simulink model "FullCardioLabModel"  (R2023b)
settings: Solver=FixedStepDiscrete  StartTime=0.0  StopTime=param_sim_time  FixedStep=1/fs  MaxStep=1/fs  RelTol=1e-3
undefined symbols (not defined in the file): analyses, fdesignblkfcn, fs, gcbh, param_tot_samples
libraries: dspstat3 x13, SCGAnalysis_SignalGenerationLib x2
(part 4 of 20)

== system FullCardioLabModel/ECG Preprocessing/Enabled ECG Preprocessing Subsystem/ECG Filtfiltering/Bandpass Filter 2 ==
  In : Inport
  Generated Filter Block : DiscreteFir  Tag=BlockMethodSubSystem  Coefficients=[-0.00679485432608760258 -0.00368052369966220989 0.00854312547844450834 -0.00080100055038292311 0.00372672989233903233 -0.000414423493004983272 0.00116500696533589489 -0.00068747703460298674 -0.00013687627970678594 -0.000908036536334603768 -0.000644757715485386033 -0.000872603667353300666 -0.000649980563873023558 -0.000610089182523331809 -0.00038439095041600032 -0.00024106878235529626 -4.03649627099907346e-05 0.000102557079219553864 0.000239825065708428893 0.000323758429883300614 0.000376057404680168019 0.000381073126084808557 0.000351986827882749646 0.000288970153653461583 0.000203557617554966464 0.000103021925348629849 -2.14972891546076422e-06 -0.000103131395606973747 -0.000191913507308220108 -0.000261698858359729039 -0.000308472416490167939 -0.000329303004746908082 -0.000324728524771220875 -0.000295994179250205389 -0.000247522226025559291 -0.000183683342227257597 -0.000111268997009052553 -3.58593887764172993e-05 3.54498621996451069e-05 9.77683410380052935e-05 0.000145703863758933665 0.000176655825985935067 0.000188094350365417429 0.000180492814203296045 0.000154473500745000095 0.000113756327285604027 6.12602210639520489e-05 1.57243384404888854e-06 -6.12830471515304854e-05 -0.000118905673343270871 -0.000166443476187149288 -0.000205625815666153269 -0.000238031351439175516 -0.000249070759457461599 -0.000232083552430289238 -0.000205754295833784494 -0.000181898702706739611 -0.0001407218603657792 -8.35522273306556451e-05 -3.21996516028640674e-05 1.7278285931823638e-05 6.81716454841805052e-05 9.80963555024212468e-05 0.000114282258451226405 0.000125390720583284248 0.000115578716749255295 9.38842976059089761e-05 6.87092823481379888e-05 2.48553026108045532e-05 -2.17355756601703342e-05 -6.75971265676663242e-05 -0.000120182111292099338 -0.000160508422265174448 -0.000191657601357176212 -0.000216576988296063457 -0.00021931111999210691 -0.000215024561640978211 -0.000197445525101160854 -0.000164771250432415092 -0.000131410053958377849 -8.71464649119211714e-05 -4.22248400762013188e-05 -2.55187176720146705e-06 3.98401007686889031e-05 6.70160005196594532e-05 8.85649928240380709e-05 9.79022940505013271e-05 9.01099694726976237e-05 7.60411656456247117e-05 4.47157145500393243e-05 7.64412579202713784e-06 -3.41205371522478645e-05 -8.26469602656201477e-05 -0.000122462466866380266 -0.000163942006908490364 -0.000192450425008703106 -0.00021198533578391723 -0.000221725958061418457 -0.000214264856837328933 -0.000201133393186481407 -0.000173112614868433816 -0.000139284113164017806 -9.91911991007083521e-05 -5.35014581152537346e-05 -1.66145969408442357e-05 2.24701480311693537e-05 5.10282875995192933e-05 7.46380231078692279e-05 8.15963671632117496e-05 7.39608989028757761e-05 6.0706597352138177e-05 3.18412262523817138e-05 -2.42321911527576506e-06 -4.59521245665078348e-05 -8.89644740066970632e-05 -0.000133478940391839891 -0.000174761594434663794 -0.000201676761858123299 -0.000225431470491829934 -0.000231411914244697713 -0.0002291228016563979 -0.000212057881694176551 -0.000187564945378138249 -0.000151900580862694972 -0.000109968801817303811 -6.93206759645438543e-05 -2.35100770337276738e-05 1.12536348097588912e-05 4.23852216138695436e-05 6.13447585404637184e-05 6.93324050786263017e-05 6.47625896664805482e-05 4.82724081093188285e-05 2.24506769099194001e-05 -1.6204546713455065e-05 -5.46536524933584976e-05 -0.000103747419230983487 -0.00014506639579119971 -0.000187106115664925236 -0.000218555841549362094 -0.000240824987275647272 -0.000250230000792608053 -0.000247129096173642087 -0.00023153260668738786 -0.000203244239201745401 -0.000169336212688825312 -0.000124006092535268773 -8.21474781826332586e-05 -3.55642321516080979e-05 2.33768767351631586e-06 3.46530747321792344e-05 5.58866889668884501e-05 6.36863963294788925e-05 5.90396372207047251e-05 4.07361313906464548e-05 1.27631651658388758e-05 -2.80294254426716e-05 -7.10729581908008736e-05 -0.000121861727445029294 -0.000162876017395040626 -0.000207719395348772472 -0.00023814974876393749 -0.000263249857604426994 ...(+45428 chars)]  InputProcessing=Columns as channels (frame based)
  Out : Outport  VectorParamsAs1DForOutWhenUnconnected=off
  wires:
  Generated Filter Block/1 -> Out/1
  In/1 -> Generated Filter Block/1
